simulink subsystem "BackwardAccConverter"  (R2023a)
settings: Solver=VariableStepAuto  StartTime=0.0  StopTime=10.0  RelTol=1e-3
undefined symbols (not defined in the file): i_gear, i_rail
settings Model: Creator=ПК  LastModifiedBy=ПК

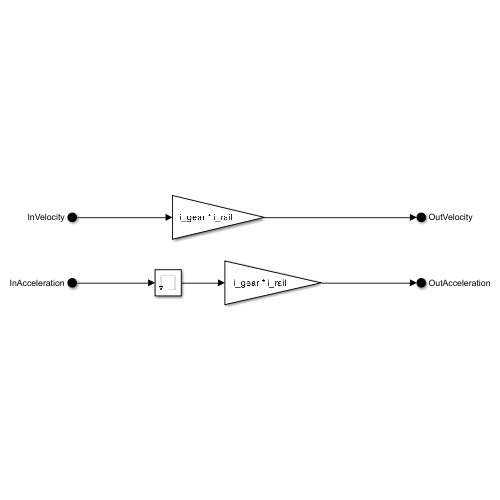
[thumbnail: Simulink's stored preview of the top-level diagram]
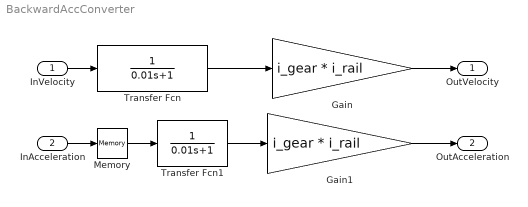
== system BackwardAccConverter ==
  InVelocity : Inport
  InAcceleration : Inport  Port=2
  Gain : Gain  Gain=i_gear * i_rail
  Gain1 : Gain  Gain=i_gear * i_rail
  Memory : Memory
  Transfer Fcn : TransferFcn  Denominator=[0.01 1]
  Transfer Fcn1 : TransferFcn  Denominator=[0.01 1]
  OutVelocity : Outport
  OutAcceleration : Outport  Port=2
  wires:
  InAcceleration/1 -> Memory/1
  Gain1/1 -> OutAcceleration/1
  Gain/1 -> OutVelocity/1
  Memory/1 -> Transfer Fcn1/1
  InVelocity/1 -> Transfer Fcn/1
  Transfer Fcn/1 -> Gain/1
  Transfer Fcn1/1 -> Gain1/1
